simulink model "functionexample"  (R2024b)
settings: Solver=FixedStepAuto  StartTime=0.0  StopTime=10.0  MaxStep=0.1  RelTol=1e-3  EnableMultiTasking=on
libraries: stm32blockslib x2
settings Model: STM32="{\"UARTRead\":[{\"ID\":\"untitled:3\"},{\"ID\":\"functionexample:3\"}],\"UARTWrite\":[{\"ID\":\"untitled:4\"},{\"ID\":\"functionexample:4\"}]}"  Creator=mivia  LastModifiedBy=mivia
settings OptimizationCC: DefaultParameterBehavior=Inlined  EnhancedBackFolding=on  PassReuseOutputArgsAs=Individual arguments  ZeroExternalMemoryAtStartup=off  ZeroInternalMemoryAtStartup=off  MaxStackSize=512  OptimizeBlockOrder=speed  DifferentSizesBufferReuse=on  OptimizationCustomize=off  EfficientTunableParamExpr=on
settings DebuggingCC: ParameterTunabilityLossMsg=error
settings HardwareCC: ProdBitPerPointer=32  ProdBitPerSizeT=32  ProdBitPerPtrDiffT=32  ProdLargestAtomicInteger=Long  ProdLargestAtomicFloat=Double  ProdWordSize=32  ProdLongLongMode=on  ProdHWDeviceType=ARM Compatible->ARM Cortex-M
settings RTWCC: Description=Embedded Coder  SystemTargetFile=ert.tlc  HardwareBoard=STM32G4xx Based  TemplateMakefile=ert_default_tmf  Toolchain=GNU Tools for ARM Embedded Processors
settings CodeAppCC: ForceParamTrailComments=on  IgnoreCustomStorageClasses=off  OperatorAnnotations=on  SimulinkDataObjDesc=on  SFDataObjDesc=on  InsertBlockDesc=on
settings ERTTargetCC: TargetLangStandard=C99 (ISO)  CodeReplacementLibrary=ARM Cortex-M  SupportVariableSizeSignals=on  ExtModeTransport=3  ExtModeStaticAlloc=on  ExtModeStaticAllocSize=2048  ExtModeMexFile=ext_xcp  ExtModeIntrfLevel=Level2 - Open

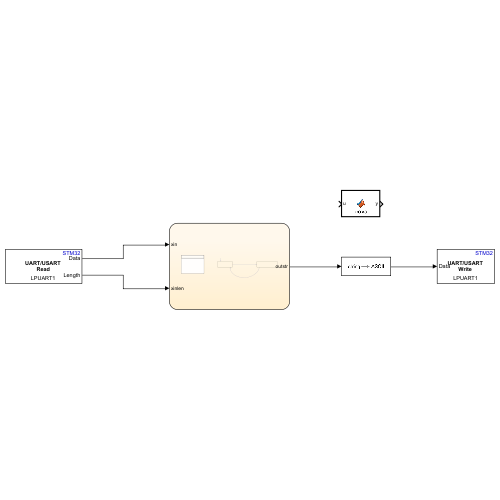
[thumbnail: Simulink's stored preview of the top-level diagram]
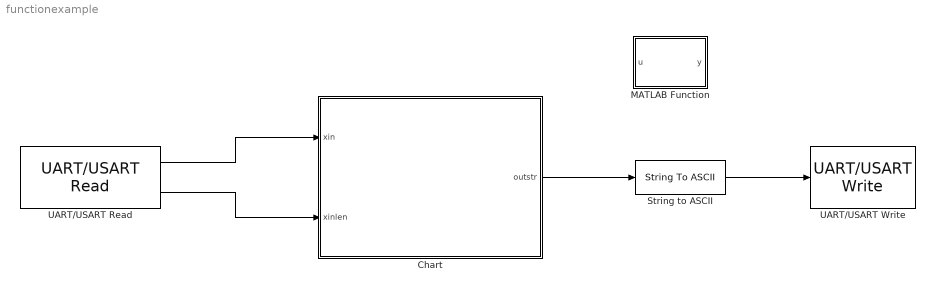
== system functionexample ==
  Chart : Stateflow chart  TreatAsAtomicUnit=on
  MATLAB Function : MATLAB Function  TreatAsAtomicUnit=on
  String to ASCII : StringToASCII  OutputVectorSize=120
  UART/USART Read : stm32blockslib/UART//USART Read  UARTModule=LPUART1  DataType=uint8  DataLength=1  BlockingMode=off  BlockingTimeout=0.1  OutputLength=on  OutputStatus=off  SampleTime=-1
      settings: LibrarySourceBlock=stm32g4xxblockslib/UART//USART Read
  UART/USART Write : stm32blockslib/UART//USART Write  UARTModule=LPUART1  LengthOfDataToSend=off  BlockingMode=off  BlockingTimeout=0.1  OutputStatus=off
      settings: LibrarySourceBlock=stm32g4xxblockslib/UART//USART Write
  wires:
  UART/USART Read/1 -> Chart/1(xin)
  UART/USART Read/2 -> Chart/2(xinlen)
  Chart/1(outstr) -> String to ASCII/1
  String to ASCII/1 -> UART/USART Write/1

== matlab function functionexample/MATLAB Function ==
  data: u input; y output
function y = prova(u)

y = zeros(127)
z = convertStringsToChars(u)
l = min(length(z),length(y));
for i = 1:l
   y(i) = z(i);
end

end

== stateflow chart functionexample/Chart ==
  state PRINT
    en: outstr = prepareMenu
    du: outstr = ""
  state LEDON
    en: outstr = "Led acceso" + newline;
    du: outstr = ""
  (default) -> PRINT
  PRINT -> LEDON : [xinlen > 0 && xin == '1']
  LEDON -> PRINT : after(5, sec)
  data: outString function_output; xin input; outstr output string; xinlen input
  function outString = prepareMenu:
    | function outString = prepareMenu
    | 
    | outString = "Cosa vuoi fare?" + newline + ...
    |     "1. Accendere un led" + newline + ...
    |     "2. Azionare il motore" + newline + ...
    |     "3. Riavviare il sistema" + newline;
    | 
    | end
